simulink model "gm_ZynqBF_2tx_fpga"  (R2018b)
settings: Solver=FixedStepDiscrete  StartTime=0.0  StopTime=10.0  FixedStep=(1/420e3)/128  RelTol=1e-3
undefined symbols (not defined in the file or in its folder): a, b, c
libraries: hdlsllib x873, simulink x349
(part 7 of 40)

== system gm_ZynqBF_2tx_fpga/channel_estimator/peakdetect_ch2/peak_fsm ==
  t_cross : Inport  OutDataTypeStr=boolean  PortDimensions=1  SampleTime=1.86011904761905e-08
  cnt_end : Inport  Port=2  OutDataTypeStr=boolean  PortDimensions=1  SampleTime=1.86011904761905e-08
  Compare To Constant : simulink/Logic and Bit Operations/Compare To Constant  relop===  const=fi(0,0,8,0,'hex','01')  OutDataTypeStr=boolean
  Compare To Constant1 : simulink/Logic and Bit Operations/Compare To Constant  relop===  const=fi(0,0,8,0,'hex','00')  OutDataTypeStr=boolean
  Compare To Constant2 : simulink/Logic and Bit Operations/Compare To Constant  relop===  const=fi(0,0,8,0,'hex','02')  OutDataTypeStr=boolean
  HDL Counter : hdlsllib/Sources/HDL Counter  CountType=Count limited  CountInit=double(0)  CountStep=double(1)  CountMax=double(3)  CountFromType=Initial value  CountFrom=double(0)  CountResetPort=off  CountLoadPort=off  CountEnbPort=on  CountDirPort=off  CountDataType=Unsigned  CountWordLen=8  CountFracLen=0  CountSampTime=1.86011904761905e-08
      settings: SourceProductBaseCode=HD
  Logical Operator : Logic  AllPortsSameDT=off  OutDataTypeStr=boolean  SampleTime=1.86011904761905e-08
  Logical Operator1 : Logic  Operator=OR  Inputs=3  AllPortsSameDT=off  OutDataTypeStr=boolean  SampleTime=1.86011904761905e-08
  scan_peak : Outport
  peak_found : Outport  Port=2
  wires:
  t_cross/1 -> Logical Operator/1
  cnt_end/1 -> Logical Operator1/2
  Compare To Constant/1 -> scan_peak/1
  Compare To Constant1/1 -> Logical Operator/2
  Compare To Constant2/1 -> Logical Operator1/1, peak_found/1
  HDL Counter/1 -> Compare To Constant2/1, Compare To Constant1/1, Compare To Constant/1
  Logical Operator/1 -> Logical Operator1/3
  Logical Operator1/1 -> HDL Counter/1

== system gm_ZynqBF_2tx_fpga/channel_estimator/peakdetect_ch2/running_max ==
  din : Inport  OutDataTypeStr=fixdt(1, 32, 16)  PortDimensions=1  SampleTime=1.86011904761905e-08
  en : Inport  Port=2  OutDataTypeStr=boolean  PortDimensions=1  SampleTime=1.86011904761905e-08
  rst : Inport  Port=3  OutDataTypeStr=boolean  PortDimensions=1  SampleTime=1.86011904761905e-08
  Constant : Constant  Value=0  OutDataTypeStr=fixdt(1, 32, 16)  SampleTime=-1
  Delay4 : Delay  DelayLength=double(1)  InitialCondition=0  InputProcessing=Inherited  SampleTime=1.86011904761905e-08
  Relational Operator : RelationalOperator  Operator=>  OutDataTypeStr=boolean  SampleTime=1.86011904761905e-08  RndMeth=Nearest
  reset_max : Switch  Criteria=u2 ~= 0  Threshold=double(0)  OutDataTypeStr=fixdt(1, 32, 16)  SampleTime=1.86011904761905e-08
  store_max : Switch  Criteria=u2 ~= 0  Threshold=double(0)  OutDataTypeStr=fixdt(1, 32, 16)  SampleTime=1.86011904761905e-08
  update_max : Logic  AllPortsSameDT=off  OutDataTypeStr=boolean  SampleTime=1.86011904761905e-08
  new_max : Outport
  max_val : Outport  Port=2
  wires:
  din/1 -> store_max/1, Relational Operator/1
  en/1 -> update_max/1
  rst/1 -> reset_max/2
  Constant/1 -> reset_max/1
  Delay4/1 -> store_max/3, Relational Operator/2, max_val/1
  Relational Operator/1 -> update_max/2
  reset_max/1 -> Delay4/1
  store_max/1 -> reset_max/3
  update_max/1 -> store_max/2, new_max/1

== system gm_ZynqBF_2tx_fpga/channel_estimator/peakdetect_ch2/store_index ==
  din : Inport  OutDataTypeStr=int16  PortDimensions=1  SampleTime=1.86011904761905e-08
  update : Inport  Port=2  OutDataTypeStr=boolean  PortDimensions=1  SampleTime=1.86011904761905e-08
  Delay{1..2,4..5} (4 alike) : Delay  DelayLength=double(1)  InitialCondition=0  InputProcessing=Inherited  SampleTime=1.86011904761905e-08
  Switch : Switch  Criteria=u2 ~= 0  Threshold=double(0)  OutDataTypeStr=int16  SampleTime=1.86011904761905e-08
  dout : Outport
  wires:
  din/1 -> Delay2/1
  update/1 -> Delay1/1
  Delay1/1 -> Switch/2
  Delay2/1 -> Switch/1
  Delay4/1 -> dout/1
  Delay5/1 -> Switch/3
  Switch/1 -> Delay5/1, Delay4/1

== system gm_ZynqBF_2tx_fpga/channel_estimator/ram_rd_counter/select_inputs ==
  en1 : Inport  OutDataTypeStr=boolean  PortDimensions=1  SampleTime=1.86011904761905e-08
  en2 : Inport  Port=2  OutDataTypeStr=boolean  PortDimensions=1  SampleTime=1.86011904761905e-08
  in1 : Inport  Port=3  OutDataTypeStr=fixdt(0, 15, 0)  PortDimensions=1  SampleTime=1.86011904761905e-08
  in2 : Inport  Port=4  OutDataTypeStr=fixdt(0, 15, 0)  PortDimensions=1  SampleTime=1.86011904761905e-08
  select_inputs : MATLAB Function  TreatAsAtomicUnit=on
  y : Outport
  wires:
  en1/1 -> select_inputs/1(en1)
  en2/1 -> select_inputs/2(en2)
  in1/1 -> select_inputs/3(in1)
  in2/1 -> select_inputs/4(in2)
  select_inputs/1(y) -> y/1

== system gm_ZynqBF_2tx_fpga/channel_estimator/ch_est/calc_inverse/HDL Reciprocal ==
  In1 : Inport
  Delay1 : Delay  DelayLength=1  InputProcessing=Inherited
  Delay2 : Delay  DelayLength=10  InputProcessing=Inherited
  HDL Reciprocal : Reciprocal  NumberOfIterations=5  SampleTime=1.86011904761905e-08
  Out1 : Outport
  wires:
  In1/1 -> Delay1/1
  Delay1/1 -> HDL Reciprocal/1
  HDL Reciprocal/1 -> Delay2/1
  Delay2/1 -> Out1/1

== system gm_ZynqBF_2tx_fpga/channel_estimator/peakdetect_ch1/correlator1/all_u ==
  u : Inport  OutDataTypeStr=boolean  PortDimensions=[8]  SampleTime=1.86011904761905e-08
  all_u : MATLAB Function  TreatAsAtomicUnit=on
  y : Outport
  wires:
  u/1 -> all_u/1(u)
  all_u/1(y) -> y/1

== system gm_ZynqBF_2tx_fpga/channel_estimator/peakdetect_ch1/correlator1/all_u1 ==
  u : Inport  OutDataTypeStr=boolean  PortDimensions=[8]  SampleTime=1.86011904761905e-08
  all_u : MATLAB Function  TreatAsAtomicUnit=on
  y : Outport
  wires:
  all_u/1(y) -> y/1
  u/1 -> all_u/1(u)

== system gm_ZynqBF_2tx_fpga/channel_estimator/peakdetect_ch1/correlator1/correlation_config ==
  rst : Inport  OutDataTypeStr=boolean  PortDimensions=1  SampleTime=1.86011904761905e-08
  vin : Inport  Port=2  OutDataTypeStr=boolean  PortDimensions=1  SampleTime=1.86011904761905e-08
  Bit Slice : hdlsllib/Logic and Bit Operations/Bit Slice  lidx=double(14)  ridx=double(6)
  Delay{1..2,4..5} (4 alike) : Delay  DelayLength=double(1)  InitialCondition=0  InputProcessing=Inherited  SampleTime=1.86011904761905e-08
  Delay6 : Delay  DelayLength=double(3)  InitialCondition=0  InputProcessing=Inherited  SampleTime=1.86011904761905e-08
  correlation_count : hdlsllib/Sources/HDL Counter  CountType=Free running  CountInit=double(32767)  CountStep=double(1)  CountMax=25  CountFromType=Initial value  CountFrom=double(32767)  CountResetPort=on  CountLoadPort=off  CountEnbPort=on  CountDirPort=off  CountDataType=Unsigned  CountWordLen=15  CountFracLen=0  CountSampTime=1.86011904761905e-08
      settings: SourceProductBaseCode=HD
  shift_count : hdlsllib/Sources/HDL Counter  CountType=Free running  CountInit=double(63)  CountStep=double(1)  CountMax=25  CountFromType=Initial value  CountFrom=double(63)  CountResetPort=on  CountLoadPort=off  CountEnbPort=on  CountDirPort=off  CountDataType=Unsigned  CountWordLen=6  CountFracLen=0  CountSampTime=1.86011904761905e-08
      settings: SourceProductBaseCode=HD
  addr : Outport
  shift : Outport  Port=2
  vout : Outport  Port=3
  wires:
  rst/1 -> Delay4/1
  vin/1 -> Delay1/1
  Bit Slice/1 -> Delay2/1
  Delay1/1 -> shift_count/2, correlation_count/2, Delay6/1
  Delay2/1 -> addr/1
  Delay4/1 -> shift_count/1, correlation_count/1
  Delay5/1 -> shift/1
  Delay6/1 -> vout/1
  correlation_count/1 -> Bit Slice/1
  shift_count/1 -> Delay5/1

== system gm_ZynqBF_2tx_fpga/channel_estimator/peakdetect_ch1/correlator1/correlator_en ==
  valid : Inport  OutDataTypeStr=boolean  PortDimensions=1  SampleTime=1.86011904761905e-08
  done : Inport  Port=2  OutDataTypeStr=boolean  PortDimensions=1  SampleTime=1.86011904761905e-08
  addri : Inport  Port=3  OutDataTypeStr=fixdt(0, 9, 0)  PortDimensions=1  SampleTime=1.86011904761905e-08
  Compare To Constant : simulink/Logic and Bit Operations/Compare To Constant  relop===  const=fi(0,0,6,0,'hex','01')  OutDataTypeStr=boolean
  Delay1 : Delay  DelayLength=double(1)  InitialCondition=0  InputProcessing=Inherited  SampleTime=1.86011904761905e-08
  Delay2 : Delay  DelayLength=double(1)  InitialCondition=0  InputProcessing=Inherited  SampleTime=1.86011904761905e-08
  Delay3 : Delay  DelayLength=double(1)  InitialCondition=0  InputProcessing=Inherited  SampleTime=1.86011904761905e-08
  Sum : Sum  AccumDataTypeStr=fixdt(0, 10, 0)  OutDataTypeStr=fixdt(0, 10, 0)  SampleTime=1.86011904761905e-08
  corr_addr : hdlsllib/Sources/HDL Counter  CountType=Count limited  CountInit=double(0)  CountStep=double(1)  CountMax=double(63)  CountFromType=Initial value  CountFrom=double(0)  CountResetPort=on  CountLoadPort=off  CountEnbPort=on  CountDirPort=off  CountDataType=Unsigned  CountWordLen=6  CountFracLen=0  CountSampTime=1.86011904761905e-08
      settings: SourceProductBaseCode=HD
  corr_state : hdlsllib/Sources/HDL Counter  CountType=Count limited  CountInit=double(0)  CountStep=double(1)  CountMax=double(1)  CountFromType=Initial value  CountFrom=double(0)  CountResetPort=on  CountLoadPort=off  CountEnbPort=on  CountDirPort=off  CountDataType=Unsigned  CountWordLen=6  CountFracLen=0  CountSampTime=1.86011904761905e-08
      settings: SourceProductBaseCode=HD
  start : Outport
  en : Outport  Port=2
  gs_addr : Outport  Port=3
  rx_addr : Outport  Port=4
  wires:
  valid/1 -> corr_addr/1, Delay1/1
  done/1 -> corr_state/1
  addri/1 -> Sum/2
  Compare To Constant/1 -> Delay2/1
  Delay1/1 -> corr_state/2, Delay3/1
  Delay2/1 -> corr_addr/2, en/1
  Delay3/1 -> start/1
  Sum/1 -> rx_addr/1
  corr_addr/1 -> Sum/1, gs_addr/1
  corr_state/1 -> Compare To Constant/1

== system gm_ZynqBF_2tx_fpga/channel_estimator/peakdetect_ch1/correlator1/correlator_i_instance1 ==
  rx : Inport  OutDataTypeStr=fixdt(1, 16, 15)  PortDimensions=1  SampleTime=1.86011904761905e-08
  gs : Inport  Port=2  OutDataTypeStr=fixdt(1, 16, 15)  PortDimensions=1  SampleTime=1.86011904761905e-08
  start : Inport  Port=3  OutDataTypeStr=boolean  PortDimensions=1  SampleTime=1.86011904761905e-08
  vin : Inport  Port=4  OutDataTypeStr=boolean  PortDimensions=1  SampleTime=1.86011904761905e-08
  Compare To Constant1 : simulink/Logic and Bit Operations/Compare To Constant  relop===  const=fi(0,0,7,0,'hex','3f')  OutDataTypeStr=boolean
  Constant : Constant  Value=0  OutDataTypeStr=fixdt(1, 32, 16)  SampleTime=-1
  Constant1 : Constant  Value=0  OutDataTypeStr=fixdt(1, 16, 15)  SampleTime=-1
  Delay1 : Delay  DelayLength=double(1)  InitialCondition=0  InputProcessing=Inherited  SampleTime=1.86011904761905e-08
  HDL Counter : hdlsllib/Sources/HDL Counter  CountType=Free running  CountInit=double(0)  CountStep=double(1)  CountMax=25  CountFromType=Initial value  CountFrom=double(0)  CountResetPort=on  CountLoadPort=off  CountEnbPort=on  CountDirPort=off  CountDataType=Unsigned  CountWordLen=7  CountFracLen=0  CountSampTime=1.86011904761905e-08
      settings: SourceProductBaseCode=HD
  Multiply-Add : hdlsllib/HDL Operations/Multiply-Add  Function=c+(a.*b)  datatype=fixdt(1, 32, 16)  DoSatur=off  FMA=off
      settings: SourceProductName=HDL Coder  SourceProductBaseCode=HD
  Switch : Switch  Criteria=u2 ~= 0  Threshold=double(0)  OutDataTypeStr=fixdt(1, 32, 16)  SampleTime=1.86011904761905e-08
  Switch1 : Switch  Criteria=u2 ~= 0  Threshold=double(0)  OutDataTypeStr=fixdt(1, 16, 15)  SampleTime=1.86011904761905e-08
  Switch2 : Switch  Criteria=u2 ~= 0  Threshold=double(0)  OutDataTypeStr=fixdt(1, 16, 15)  SampleTime=1.86011904761905e-08
  dout : Outport
  vout : Outport  Port=2
  wires:
  Switch2/1 -> Multiply-Add/2
  Switch1/1 -> Multiply-Add/1
  Multiply-Add/1 -> dout/1, Delay1/1
  HDL Counter/1 -> Compare To Constant1/1
  Constant1/1 -> Switch1/3, Switch2/3
  Constant/1 -> Switch/1
  Compare To Constant1/1 -> vout/1
  rx/1 -> Switch1/1
  gs/1 -> Switch2/1
  start/1 -> HDL Counter/1, Switch/2
  vin/1 -> Switch1/2, Switch2/2, HDL Counter/2
  Delay1/1 -> Switch/3
  Switch/1 -> Multiply-Add/3

== system gm_ZynqBF_2tx_fpga/channel_estimator/peakdetect_ch1/correlator1/correlator_i_instance10 ==
  rx : Inport  OutDataTypeStr=fixdt(1, 16, 15)  PortDimensions=1  SampleTime=1.86011904761905e-08
  gs : Inport  Port=2  OutDataTypeStr=fixdt(1, 16, 15)  PortDimensions=1  SampleTime=1.86011904761905e-08
  start : Inport  Port=3  OutDataTypeStr=boolean  PortDimensions=1  SampleTime=1.86011904761905e-08
  vin : Inport  Port=4  OutDataTypeStr=boolean  PortDimensions=1  SampleTime=1.86011904761905e-08
  Compare To Constant1 : simulink/Logic and Bit Operations/Compare To Constant  relop===  const=fi(0,0,7,0,'hex','3f')  OutDataTypeStr=boolean
  Constant : Constant  Value=0  OutDataTypeStr=fixdt(1, 32, 16)  SampleTime=-1
  Constant1 : Constant  Value=0  OutDataTypeStr=fixdt(1, 16, 15)  SampleTime=-1
  Delay1 : Delay  DelayLength=double(1)  InitialCondition=0  InputProcessing=Inherited  SampleTime=1.86011904761905e-08
  HDL Counter : hdlsllib/Sources/HDL Counter  CountType=Free running  CountInit=double(0)  CountStep=double(1)  CountMax=25  CountFromType=Initial value  CountFrom=double(0)  CountResetPort=on  CountLoadPort=off  CountEnbPort=on  CountDirPort=off  CountDataType=Unsigned  CountWordLen=7  CountFracLen=0  CountSampTime=1.86011904761905e-08
      settings: SourceProductBaseCode=HD
  Multiply-Add : hdlsllib/HDL Operations/Multiply-Add  Function=c+(a.*b)  datatype=fixdt(1, 32, 16)  DoSatur=off  FMA=off
      settings: SourceProductName=HDL Coder  SourceProductBaseCode=HD
  Switch : Switch  Criteria=u2 ~= 0  Threshold=double(0)  OutDataTypeStr=fixdt(1, 32, 16)  SampleTime=1.86011904761905e-08
  Switch1 : Switch  Criteria=u2 ~= 0  Threshold=double(0)  OutDataTypeStr=fixdt(1, 16, 15)  SampleTime=1.86011904761905e-08
  Switch2 : Switch  Criteria=u2 ~= 0  Threshold=double(0)  OutDataTypeStr=fixdt(1, 16, 15)  SampleTime=1.86011904761905e-08
  dout : Outport
  vout : Outport  Port=2
  wires:
  Switch/1 -> Multiply-Add/3
  Delay1/1 -> Switch/3
  vin/1 -> HDL Counter/2, Switch2/2, Switch1/2
  start/1 -> Switch/2, HDL Counter/1
  gs/1 -> Switch2/1
  rx/1 -> Switch1/1
  Compare To Constant1/1 -> vout/1
  Constant/1 -> Switch/1
  Constant1/1 -> Switch2/3, Switch1/3
  HDL Counter/1 -> Compare To Constant1/1
  Multiply-Add/1 -> Delay1/1, dout/1
  Switch1/1 -> Multiply-Add/1
  Switch2/1 -> Multiply-Add/2

== system gm_ZynqBF_2tx_fpga/channel_estimator/peakdetect_ch1/correlator1/correlator_i_instance11 ==
  rx : Inport  OutDataTypeStr=fixdt(1, 16, 15)  PortDimensions=1  SampleTime=1.86011904761905e-08
  gs : Inport  Port=2  OutDataTypeStr=fixdt(1, 16, 15)  PortDimensions=1  SampleTime=1.86011904761905e-08
  start : Inport  Port=3  OutDataTypeStr=boolean  PortDimensions=1  SampleTime=1.86011904761905e-08
  vin : Inport  Port=4  OutDataTypeStr=boolean  PortDimensions=1  SampleTime=1.86011904761905e-08
  Compare To Constant1 : simulink/Logic and Bit Operations/Compare To Constant  relop===  const=fi(0,0,7,0,'hex','3f')  OutDataTypeStr=boolean
  Constant : Constant  Value=0  OutDataTypeStr=fixdt(1, 32, 16)  SampleTime=-1
  Constant1 : Constant  Value=0  OutDataTypeStr=fixdt(1, 16, 15)  SampleTime=-1
  Delay1 : Delay  DelayLength=double(1)  InitialCondition=0  InputProcessing=Inherited  SampleTime=1.86011904761905e-08
  HDL Counter : hdlsllib/Sources/HDL Counter  CountType=Free running  CountInit=double(0)  CountStep=double(1)  CountMax=25  CountFromType=Initial value  CountFrom=double(0)  CountResetPort=on  CountLoadPort=off  CountEnbPort=on  CountDirPort=off  CountDataType=Unsigned  CountWordLen=7  CountFracLen=0  CountSampTime=1.86011904761905e-08
      settings: SourceProductBaseCode=HD
  Multiply-Add : hdlsllib/HDL Operations/Multiply-Add  Function=c+(a.*b)  datatype=fixdt(1, 32, 16)  DoSatur=off  FMA=off
      settings: SourceProductName=HDL Coder  SourceProductBaseCode=HD
  Switch : Switch  Criteria=u2 ~= 0  Threshold=double(0)  OutDataTypeStr=fixdt(1, 32, 16)  SampleTime=1.86011904761905e-08
  Switch1 : Switch  Criteria=u2 ~= 0  Threshold=double(0)  OutDataTypeStr=fixdt(1, 16, 15)  SampleTime=1.86011904761905e-08
  Switch2 : Switch  Criteria=u2 ~= 0  Threshold=double(0)  OutDataTypeStr=fixdt(1, 16, 15)  SampleTime=1.86011904761905e-08
  dout : Outport
  vout : Outport  Port=2
  wires:
  Switch/1 -> Multiply-Add/3
  Delay1/1 -> Switch/3
  vin/1 -> HDL Counter/2, Switch2/2, Switch1/2
  start/1 -> Switch/2, HDL Counter/1
  gs/1 -> Switch2/1
  rx/1 -> Switch1/1
  Compare To Constant1/1 -> vout/1
  Constant/1 -> Switch/1
  Constant1/1 -> Switch2/3, Switch1/3
  HDL Counter/1 -> Compare To Constant1/1
  Multiply-Add/1 -> Delay1/1, dout/1
  Switch1/1 -> Multiply-Add/1
  Switch2/1 -> Multiply-Add/2

== system gm_ZynqBF_2tx_fpga/channel_estimator/peakdetect_ch1/correlator1/correlator_i_instance12 ==
  rx : Inport  OutDataTypeStr=fixdt(1, 16, 15)  PortDimensions=1  SampleTime=1.86011904761905e-08
  gs : Inport  Port=2  OutDataTypeStr=fixdt(1, 16, 15)  PortDimensions=1  SampleTime=1.86011904761905e-08
  start : Inport  Port=3  OutDataTypeStr=boolean  PortDimensions=1  SampleTime=1.86011904761905e-08
  vin : Inport  Port=4  OutDataTypeStr=boolean  PortDimensions=1  SampleTime=1.86011904761905e-08
  Compare To Constant1 : simulink/Logic and Bit Operations/Compare To Constant  relop===  const=fi(0,0,7,0,'hex','3f')  OutDataTypeStr=boolean
  Constant : Constant  Value=0  OutDataTypeStr=fixdt(1, 32, 16)  SampleTime=-1
  Constant1 : Constant  Value=0  OutDataTypeStr=fixdt(1, 16, 15)  SampleTime=-1
  Delay1 : Delay  DelayLength=double(1)  InitialCondition=0  InputProcessing=Inherited  SampleTime=1.86011904761905e-08
  HDL Counter : hdlsllib/Sources/HDL Counter  CountType=Free running  CountInit=double(0)  CountStep=double(1)  CountMax=25  CountFromType=Initial value  CountFrom=double(0)  CountResetPort=on  CountLoadPort=off  CountEnbPort=on  CountDirPort=off  CountDataType=Unsigned  CountWordLen=7  CountFracLen=0  CountSampTime=1.86011904761905e-08
      settings: SourceProductBaseCode=HD
  Multiply-Add : hdlsllib/HDL Operations/Multiply-Add  Function=c+(a.*b)  datatype=fixdt(1, 32, 16)  DoSatur=off  FMA=off
      settings: SourceProductName=HDL Coder  SourceProductBaseCode=HD
  Switch : Switch  Criteria=u2 ~= 0  Threshold=double(0)  OutDataTypeStr=fixdt(1, 32, 16)  SampleTime=1.86011904761905e-08
  Switch1 : Switch  Criteria=u2 ~= 0  Threshold=double(0)  OutDataTypeStr=fixdt(1, 16, 15)  SampleTime=1.86011904761905e-08
  Switch2 : Switch  Criteria=u2 ~= 0  Threshold=double(0)  OutDataTypeStr=fixdt(1, 16, 15)  SampleTime=1.86011904761905e-08
  dout : Outport
  vout : Outport  Port=2
  wires:
  Switch/1 -> Multiply-Add/3
  Delay1/1 -> Switch/3
  vin/1 -> HDL Counter/2, Switch2/2, Switch1/2
  start/1 -> Switch/2, HDL Counter/1
  gs/1 -> Switch2/1
  rx/1 -> Switch1/1
  Compare To Constant1/1 -> vout/1
  Constant/1 -> Switch/1
  Constant1/1 -> Switch2/3, Switch1/3
  HDL Counter/1 -> Compare To Constant1/1
  Multiply-Add/1 -> Delay1/1, dout/1
  Switch1/1 -> Multiply-Add/1
  Switch2/1 -> Multiply-Add/2

== system gm_ZynqBF_2tx_fpga/channel_estimator/peakdetect_ch1/correlator1/correlator_i_instance13 ==
  rx : Inport  OutDataTypeStr=fixdt(1, 16, 15)  PortDimensions=1  SampleTime=1.86011904761905e-08
  gs : Inport  Port=2  OutDataTypeStr=fixdt(1, 16, 15)  PortDimensions=1  SampleTime=1.86011904761905e-08
  start : Inport  Port=3  OutDataTypeStr=boolean  PortDimensions=1  SampleTime=1.86011904761905e-08
  vin : Inport  Port=4  OutDataTypeStr=boolean  PortDimensions=1  SampleTime=1.86011904761905e-08
  Compare To Constant1 : simulink/Logic and Bit Operations/Compare To Constant  relop===  const=fi(0,0,7,0,'hex','3f')  OutDataTypeStr=boolean
  Constant : Constant  Value=0  OutDataTypeStr=fixdt(1, 32, 16)  SampleTime=-1
  Constant1 : Constant  Value=0  OutDataTypeStr=fixdt(1, 16, 15)  SampleTime=-1
  Delay1 : Delay  DelayLength=double(1)  InitialCondition=0  InputProcessing=Inherited  SampleTime=1.86011904761905e-08
  HDL Counter : hdlsllib/Sources/HDL Counter  CountType=Free running  CountInit=double(0)  CountStep=double(1)  CountMax=25  CountFromType=Initial value  CountFrom=double(0)  CountResetPort=on  CountLoadPort=off  CountEnbPort=on  CountDirPort=off  CountDataType=Unsigned  CountWordLen=7  CountFracLen=0  CountSampTime=1.86011904761905e-08
      settings: SourceProductBaseCode=HD
  Multiply-Add : hdlsllib/HDL Operations/Multiply-Add  Function=c+(a.*b)  datatype=fixdt(1, 32, 16)  DoSatur=off  FMA=off
      settings: SourceProductName=HDL Coder  SourceProductBaseCode=HD
  Switch : Switch  Criteria=u2 ~= 0  Threshold=double(0)  OutDataTypeStr=fixdt(1, 32, 16)  SampleTime=1.86011904761905e-08
  Switch1 : Switch  Criteria=u2 ~= 0  Threshold=double(0)  OutDataTypeStr=fixdt(1, 16, 15)  SampleTime=1.86011904761905e-08
  Switch2 : Switch  Criteria=u2 ~= 0  Threshold=double(0)  OutDataTypeStr=fixdt(1, 16, 15)  SampleTime=1.86011904761905e-08
  dout : Outport
  vout : Outport  Port=2
  wires:
  Switch/1 -> Multiply-Add/3
  Delay1/1 -> Switch/3
  vin/1 -> HDL Counter/2, Switch2/2, Switch1/2
  start/1 -> Switch/2, HDL Counter/1
  gs/1 -> Switch2/1
  rx/1 -> Switch1/1
  Compare To Constant1/1 -> vout/1
  Constant/1 -> Switch/1
  Constant1/1 -> Switch2/3, Switch1/3
  HDL Counter/1 -> Compare To Constant1/1
  Multiply-Add/1 -> Delay1/1, dout/1
  Switch1/1 -> Multiply-Add/1
  Switch2/1 -> Multiply-Add/2

== system gm_ZynqBF_2tx_fpga/channel_estimator/peakdetect_ch1/correlator1/correlator_i_instance14 ==
  rx : Inport  OutDataTypeStr=fixdt(1, 16, 15)  PortDimensions=1  SampleTime=1.86011904761905e-08
  gs : Inport  Port=2  OutDataTypeStr=fixdt(1, 16, 15)  PortDimensions=1  SampleTime=1.86011904761905e-08
  start : Inport  Port=3  OutDataTypeStr=boolean  PortDimensions=1  SampleTime=1.86011904761905e-08
  vin : Inport  Port=4  OutDataTypeStr=boolean  PortDimensions=1  SampleTime=1.86011904761905e-08
  Compare To Constant1 : simulink/Logic and Bit Operations/Compare To Constant  relop===  const=fi(0,0,7,0,'hex','3f')  OutDataTypeStr=boolean
  Constant : Constant  Value=0  OutDataTypeStr=fixdt(1, 32, 16)  SampleTime=-1
  Constant1 : Constant  Value=0  OutDataTypeStr=fixdt(1, 16, 15)  SampleTime=-1
  Delay1 : Delay  DelayLength=double(1)  InitialCondition=0  InputProcessing=Inherited  SampleTime=1.86011904761905e-08
  HDL Counter : hdlsllib/Sources/HDL Counter  CountType=Free running  CountInit=double(0)  CountStep=double(1)  CountMax=25  CountFromType=Initial value  CountFrom=double(0)  CountResetPort=on  CountLoadPort=off  CountEnbPort=on  CountDirPort=off  CountDataType=Unsigned  CountWordLen=7  CountFracLen=0  CountSampTime=1.86011904761905e-08
      settings: SourceProductBaseCode=HD
  Multiply-Add : hdlsllib/HDL Operations/Multiply-Add  Function=c+(a.*b)  datatype=fixdt(1, 32, 16)  DoSatur=off  FMA=off
      settings: SourceProductName=HDL Coder  SourceProductBaseCode=HD
  Switch : Switch  Criteria=u2 ~= 0  Threshold=double(0)  OutDataTypeStr=fixdt(1, 32, 16)  SampleTime=1.86011904761905e-08
  Switch1 : Switch  Criteria=u2 ~= 0  Threshold=double(0)  OutDataTypeStr=fixdt(1, 16, 15)  SampleTime=1.86011904761905e-08
  Switch2 : Switch  Criteria=u2 ~= 0  Threshold=double(0)  OutDataTypeStr=fixdt(1, 16, 15)  SampleTime=1.86011904761905e-08
  dout : Outport
  vout : Outport  Port=2
  wires:
  Switch/1 -> Multiply-Add/3
  Delay1/1 -> Switch/3
  vin/1 -> HDL Counter/2, Switch2/2, Switch1/2
  start/1 -> Switch/2, HDL Counter/1
  gs/1 -> Switch2/1
  rx/1 -> Switch1/1
  Compare To Constant1/1 -> vout/1
  Constant/1 -> Switch/1
  Constant1/1 -> Switch2/3, Switch1/3
  HDL Counter/1 -> Compare To Constant1/1
  Multiply-Add/1 -> Delay1/1, dout/1
  Switch1/1 -> Multiply-Add/1
  Switch2/1 -> Multiply-Add/2

== system gm_ZynqBF_2tx_fpga/channel_estimator/peakdetect_ch1/correlator1/correlator_i_instance15 ==
  rx : Inport  OutDataTypeStr=fixdt(1, 16, 15)  PortDimensions=1  SampleTime=1.86011904761905e-08
  gs : Inport  Port=2  OutDataTypeStr=fixdt(1, 16, 15)  PortDimensions=1  SampleTime=1.86011904761905e-08
  start : Inport  Port=3  OutDataTypeStr=boolean  PortDimensions=1  SampleTime=1.86011904761905e-08
  vin : Inport  Port=4  OutDataTypeStr=boolean  PortDimensions=1  SampleTime=1.86011904761905e-08
  Compare To Constant1 : simulink/Logic and Bit Operations/Compare To Constant  relop===  const=fi(0,0,7,0,'hex','3f')  OutDataTypeStr=boolean
  Constant : Constant  Value=0  OutDataTypeStr=fixdt(1, 32, 16)  SampleTime=-1
  Constant1 : Constant  Value=0  OutDataTypeStr=fixdt(1, 16, 15)  SampleTime=-1
  Delay1 : Delay  DelayLength=double(1)  InitialCondition=0  InputProcessing=Inherited  SampleTime=1.86011904761905e-08
  HDL Counter : hdlsllib/Sources/HDL Counter  CountType=Free running  CountInit=double(0)  CountStep=double(1)  CountMax=25  CountFromType=Initial value  CountFrom=double(0)  CountResetPort=on  CountLoadPort=off  CountEnbPort=on  CountDirPort=off  CountDataType=Unsigned  CountWordLen=7  CountFracLen=0  CountSampTime=1.86011904761905e-08
      settings: SourceProductBaseCode=HD
  Multiply-Add : hdlsllib/HDL Operations/Multiply-Add  Function=c+(a.*b)  datatype=fixdt(1, 32, 16)  DoSatur=off  FMA=off
      settings: SourceProductName=HDL Coder  SourceProductBaseCode=HD
  Switch : Switch  Criteria=u2 ~= 0  Threshold=double(0)  OutDataTypeStr=fixdt(1, 32, 16)  SampleTime=1.86011904761905e-08
  Switch1 : Switch  Criteria=u2 ~= 0  Threshold=double(0)  OutDataTypeStr=fixdt(1, 16, 15)  SampleTime=1.86011904761905e-08
  Switch2 : Switch  Criteria=u2 ~= 0  Threshold=double(0)  OutDataTypeStr=fixdt(1, 16, 15)  SampleTime=1.86011904761905e-08
  dout : Outport
  vout : Outport  Port=2
  wires:
  Switch/1 -> Multiply-Add/3
  Delay1/1 -> Switch/3
  vin/1 -> HDL Counter/2, Switch2/2, Switch1/2
  start/1 -> Switch/2, HDL Counter/1
  gs/1 -> Switch2/1
  rx/1 -> Switch1/1
  Compare To Constant1/1 -> vout/1
  Constant/1 -> Switch/1
  Constant1/1 -> Switch2/3, Switch1/3
  HDL Counter/1 -> Compare To Constant1/1
  Multiply-Add/1 -> Delay1/1, dout/1
  Switch1/1 -> Multiply-Add/1
  Switch2/1 -> Multiply-Add/2

== system gm_ZynqBF_2tx_fpga/channel_estimator/peakdetect_ch1/correlator1/correlator_i_instance16 ==
  rx : Inport  OutDataTypeStr=fixdt(1, 16, 15)  PortDimensions=1  SampleTime=1.86011904761905e-08
  gs : Inport  Port=2  OutDataTypeStr=fixdt(1, 16, 15)  PortDimensions=1  SampleTime=1.86011904761905e-08
  start : Inport  Port=3  OutDataTypeStr=boolean  PortDimensions=1  SampleTime=1.86011904761905e-08
  vin : Inport  Port=4  OutDataTypeStr=boolean  PortDimensions=1  SampleTime=1.86011904761905e-08
  Compare To Constant1 : simulink/Logic and Bit Operations/Compare To Constant  relop===  const=fi(0,0,7,0,'hex','3f')  OutDataTypeStr=boolean
  Constant : Constant  Value=0  OutDataTypeStr=fixdt(1, 32, 16)  SampleTime=-1
  Constant1 : Constant  Value=0  OutDataTypeStr=fixdt(1, 16, 15)  SampleTime=-1
  Delay1 : Delay  DelayLength=double(1)  InitialCondition=0  InputProcessing=Inherited  SampleTime=1.86011904761905e-08
  HDL Counter : hdlsllib/Sources/HDL Counter  CountType=Free running  CountInit=double(0)  CountStep=double(1)  CountMax=25  CountFromType=Initial value  CountFrom=double(0)  CountResetPort=on  CountLoadPort=off  CountEnbPort=on  CountDirPort=off  CountDataType=Unsigned  CountWordLen=7  CountFracLen=0  CountSampTime=1.86011904761905e-08
      settings: SourceProductBaseCode=HD
  Multiply-Add : hdlsllib/HDL Operations/Multiply-Add  Function=c+(a.*b)  datatype=fixdt(1, 32, 16)  DoSatur=off  FMA=off
      settings: SourceProductName=HDL Coder  SourceProductBaseCode=HD
  Switch : Switch  Criteria=u2 ~= 0  Threshold=double(0)  OutDataTypeStr=fixdt(1, 32, 16)  SampleTime=1.86011904761905e-08
  Switch1 : Switch  Criteria=u2 ~= 0  Threshold=double(0)  OutDataTypeStr=fixdt(1, 16, 15)  SampleTime=1.86011904761905e-08
  Switch2 : Switch  Criteria=u2 ~= 0  Threshold=double(0)  OutDataTypeStr=fixdt(1, 16, 15)  SampleTime=1.86011904761905e-08
  dout : Outport
  vout : Outport  Port=2
  wires:
  Switch/1 -> Multiply-Add/3
  Delay1/1 -> Switch/3
  vin/1 -> HDL Counter/2, Switch2/2, Switch1/2
  start/1 -> Switch/2, HDL Counter/1
  gs/1 -> Switch2/1
  rx/1 -> Switch1/1
  Compare To Constant1/1 -> vout/1
  Constant/1 -> Switch/1
  Constant1/1 -> Switch2/3, Switch1/3
  HDL Counter/1 -> Compare To Constant1/1
  Multiply-Add/1 -> Delay1/1, dout/1
  Switch1/1 -> Multiply-Add/1
  Switch2/1 -> Multiply-Add/2

== system gm_ZynqBF_2tx_fpga/channel_estimator/peakdetect_ch1/correlator1/correlator_i_instance17 ==
  rx : Inport  OutDataTypeStr=fixdt(1, 16, 15)  PortDimensions=1  SampleTime=1.86011904761905e-08
  gs : Inport  Port=2  OutDataTypeStr=fixdt(1, 16, 15)  PortDimensions=1  SampleTime=1.86011904761905e-08
  start : Inport  Port=3  OutDataTypeStr=boolean  PortDimensions=1  SampleTime=1.86011904761905e-08
  vin : Inport  Port=4  OutDataTypeStr=boolean  PortDimensions=1  SampleTime=1.86011904761905e-08
  Compare To Constant1 : simulink/Logic and Bit Operations/Compare To Constant  relop===  const=fi(0,0,7,0,'hex','3f')  OutDataTypeStr=boolean
  Constant : Constant  Value=0  OutDataTypeStr=fixdt(1, 32, 16)  SampleTime=-1
  Constant1 : Constant  Value=0  OutDataTypeStr=fixdt(1, 16, 15)  SampleTime=-1
  Delay1 : Delay  DelayLength=double(1)  InitialCondition=0  InputProcessing=Inherited  SampleTime=1.86011904761905e-08
  HDL Counter : hdlsllib/Sources/HDL Counter  CountType=Free running  CountInit=double(0)  CountStep=double(1)  CountMax=25  CountFromType=Initial value  CountFrom=double(0)  CountResetPort=on  CountLoadPort=off  CountEnbPort=on  CountDirPort=off  CountDataType=Unsigned  CountWordLen=7  CountFracLen=0  CountSampTime=1.86011904761905e-08
      settings: SourceProductBaseCode=HD
  Multiply-Add : hdlsllib/HDL Operations/Multiply-Add  Function=c+(a.*b)  datatype=fixdt(1, 32, 16)  DoSatur=off  FMA=off
      settings: SourceProductName=HDL Coder  SourceProductBaseCode=HD
  Switch : Switch  Criteria=u2 ~= 0  Threshold=double(0)  OutDataTypeStr=fixdt(1, 32, 16)  SampleTime=1.86011904761905e-08
  Switch1 : Switch  Criteria=u2 ~= 0  Threshold=double(0)  OutDataTypeStr=fixdt(1, 16, 15)  SampleTime=1.86011904761905e-08
  Switch2 : Switch  Criteria=u2 ~= 0  Threshold=double(0)  OutDataTypeStr=fixdt(1, 16, 15)  SampleTime=1.86011904761905e-08
  dout : Outport
  vout : Outport  Port=2
  wires:
  Switch/1 -> Multiply-Add/3
  Delay1/1 -> Switch/3
  vin/1 -> HDL Counter/2, Switch2/2, Switch1/2
  start/1 -> Switch/2, HDL Counter/1
  gs/1 -> Switch2/1
  rx/1 -> Switch1/1
  Compare To Constant1/1 -> vout/1
  Constant/1 -> Switch/1
  Constant1/1 -> Switch2/3, Switch1/3
  HDL Counter/1 -> Compare To Constant1/1
  Multiply-Add/1 -> Delay1/1, dout/1
  Switch1/1 -> Multiply-Add/1
  Switch2/1 -> Multiply-Add/2

== system gm_ZynqBF_2tx_fpga/channel_estimator/peakdetect_ch1/correlator1/correlator_i_instance18 ==
  rx : Inport  OutDataTypeStr=fixdt(1, 16, 15)  PortDimensions=1  SampleTime=1.86011904761905e-08
  gs : Inport  Port=2  OutDataTypeStr=fixdt(1, 16, 15)  PortDimensions=1  SampleTime=1.86011904761905e-08
  start : Inport  Port=3  OutDataTypeStr=boolean  PortDimensions=1  SampleTime=1.86011904761905e-08
  vin : Inport  Port=4  OutDataTypeStr=boolean  PortDimensions=1  SampleTime=1.86011904761905e-08
  Compare To Constant1 : simulink/Logic and Bit Operations/Compare To Constant  relop===  const=fi(0,0,7,0,'hex','3f')  OutDataTypeStr=boolean
  Constant : Constant  Value=0  OutDataTypeStr=fixdt(1, 32, 16)  SampleTime=-1
  Constant1 : Constant  Value=0  OutDataTypeStr=fixdt(1, 16, 15)  SampleTime=-1
  Delay1 : Delay  DelayLength=double(1)  InitialCondition=0  InputProcessing=Inherited  SampleTime=1.86011904761905e-08
  HDL Counter : hdlsllib/Sources/HDL Counter  CountType=Free running  CountInit=double(0)  CountStep=double(1)  CountMax=25  CountFromType=Initial value  CountFrom=double(0)  CountResetPort=on  CountLoadPort=off  CountEnbPort=on  CountDirPort=off  CountDataType=Unsigned  CountWordLen=7  CountFracLen=0  CountSampTime=1.86011904761905e-08
      settings: SourceProductBaseCode=HD
  Multiply-Add : hdlsllib/HDL Operations/Multiply-Add  Function=c+(a.*b)  datatype=fixdt(1, 32, 16)  DoSatur=off  FMA=off
      settings: SourceProductName=HDL Coder  SourceProductBaseCode=HD
  Switch : Switch  Criteria=u2 ~= 0  Threshold=double(0)  OutDataTypeStr=fixdt(1, 32, 16)  SampleTime=1.86011904761905e-08
  Switch1 : Switch  Criteria=u2 ~= 0  Threshold=double(0)  OutDataTypeStr=fixdt(1, 16, 15)  SampleTime=1.86011904761905e-08
  Switch2 : Switch  Criteria=u2 ~= 0  Threshold=double(0)  OutDataTypeStr=fixdt(1, 16, 15)  SampleTime=1.86011904761905e-08
  dout : Outport
  vout : Outport  Port=2
  wires:
  Switch/1 -> Multiply-Add/3
  Delay1/1 -> Switch/3
  vin/1 -> HDL Counter/2, Switch2/2, Switch1/2
  start/1 -> Switch/2, HDL Counter/1
  gs/1 -> Switch2/1
  rx/1 -> Switch1/1
  Compare To Constant1/1 -> vout/1
  Constant/1 -> Switch/1
  Constant1/1 -> Switch2/3, Switch1/3
  HDL Counter/1 -> Compare To Constant1/1
  Multiply-Add/1 -> Delay1/1, dout/1
  Switch1/1 -> Multiply-Add/1
  Switch2/1 -> Multiply-Add/2

== system gm_ZynqBF_2tx_fpga/channel_estimator/peakdetect_ch1/correlator1/correlator_i_instance19 ==
  rx : Inport  OutDataTypeStr=fixdt(1, 16, 15)  PortDimensions=1  SampleTime=1.86011904761905e-08
  gs : Inport  Port=2  OutDataTypeStr=fixdt(1, 16, 15)  PortDimensions=1  SampleTime=1.86011904761905e-08
  start : Inport  Port=3  OutDataTypeStr=boolean  PortDimensions=1  SampleTime=1.86011904761905e-08
  vin : Inport  Port=4  OutDataTypeStr=boolean  PortDimensions=1  SampleTime=1.86011904761905e-08
  Compare To Constant1 : simulink/Logic and Bit Operations/Compare To Constant  relop===  const=fi(0,0,7,0,'hex','3f')  OutDataTypeStr=boolean
  Constant : Constant  Value=0  OutDataTypeStr=fixdt(1, 32, 16)  SampleTime=-1
  Constant1 : Constant  Value=0  OutDataTypeStr=fixdt(1, 16, 15)  SampleTime=-1
  Delay1 : Delay  DelayLength=double(1)  InitialCondition=0  InputProcessing=Inherited  SampleTime=1.86011904761905e-08
  HDL Counter : hdlsllib/Sources/HDL Counter  CountType=Free running  CountInit=double(0)  CountStep=double(1)  CountMax=25  CountFromType=Initial value  CountFrom=double(0)  CountResetPort=on  CountLoadPort=off  CountEnbPort=on  CountDirPort=off  CountDataType=Unsigned  CountWordLen=7  CountFracLen=0  CountSampTime=1.86011904761905e-08
      settings: SourceProductBaseCode=HD
  Multiply-Add : hdlsllib/HDL Operations/Multiply-Add  Function=c+(a.*b)  datatype=fixdt(1, 32, 16)  DoSatur=off  FMA=off
      settings: SourceProductName=HDL Coder  SourceProductBaseCode=HD
  Switch : Switch  Criteria=u2 ~= 0  Threshold=double(0)  OutDataTypeStr=fixdt(1, 32, 16)  SampleTime=1.86011904761905e-08
  Switch1 : Switch  Criteria=u2 ~= 0  Threshold=double(0)  OutDataTypeStr=fixdt(1, 16, 15)  SampleTime=1.86011904761905e-08
  Switch2 : Switch  Criteria=u2 ~= 0  Threshold=double(0)  OutDataTypeStr=fixdt(1, 16, 15)  SampleTime=1.86011904761905e-08
  dout : Outport
  vout : Outport  Port=2
  wires:
  Switch/1 -> Multiply-Add/3
  Delay1/1 -> Switch/3
  vin/1 -> HDL Counter/2, Switch2/2, Switch1/2
  start/1 -> Switch/2, HDL Counter/1
  gs/1 -> Switch2/1
  rx/1 -> Switch1/1
  Compare To Constant1/1 -> vout/1
  Constant/1 -> Switch/1
  Constant1/1 -> Switch2/3, Switch1/3
  HDL Counter/1 -> Compare To Constant1/1
  Multiply-Add/1 -> Delay1/1, dout/1
  Switch1/1 -> Multiply-Add/1
  Switch2/1 -> Multiply-Add/2

== system gm_ZynqBF_2tx_fpga/channel_estimator/peakdetect_ch1/correlator1/correlator_i_instance2 ==
  rx : Inport  OutDataTypeStr=fixdt(1, 16, 15)  PortDimensions=1  SampleTime=1.86011904761905e-08
  gs : Inport  Port=2  OutDataTypeStr=fixdt(1, 16, 15)  PortDimensions=1  SampleTime=1.86011904761905e-08
  start : Inport  Port=3  OutDataTypeStr=boolean  PortDimensions=1  SampleTime=1.86011904761905e-08
  vin : Inport  Port=4  OutDataTypeStr=boolean  PortDimensions=1  SampleTime=1.86011904761905e-08
  Compare To Constant1 : simulink/Logic and Bit Operations/Compare To Constant  relop===  const=fi(0,0,7,0,'hex','3f')  OutDataTypeStr=boolean
  Constant : Constant  Value=0  OutDataTypeStr=fixdt(1, 32, 16)  SampleTime=-1
  Constant1 : Constant  Value=0  OutDataTypeStr=fixdt(1, 16, 15)  SampleTime=-1
  Delay1 : Delay  DelayLength=double(1)  InitialCondition=0  InputProcessing=Inherited  SampleTime=1.86011904761905e-08
  HDL Counter : hdlsllib/Sources/HDL Counter  CountType=Free running  CountInit=double(0)  CountStep=double(1)  CountMax=25  CountFromType=Initial value  CountFrom=double(0)  CountResetPort=on  CountLoadPort=off  CountEnbPort=on  CountDirPort=off  CountDataType=Unsigned  CountWordLen=7  CountFracLen=0  CountSampTime=1.86011904761905e-08
      settings: SourceProductBaseCode=HD
  Multiply-Add : hdlsllib/HDL Operations/Multiply-Add  Function=c+(a.*b)  datatype=fixdt(1, 32, 16)  DoSatur=off  FMA=off
      settings: SourceProductName=HDL Coder  SourceProductBaseCode=HD
  Switch : Switch  Criteria=u2 ~= 0  Threshold=double(0)  OutDataTypeStr=fixdt(1, 32, 16)  SampleTime=1.86011904761905e-08
  Switch1 : Switch  Criteria=u2 ~= 0  Threshold=double(0)  OutDataTypeStr=fixdt(1, 16, 15)  SampleTime=1.86011904761905e-08
  Switch2 : Switch  Criteria=u2 ~= 0  Threshold=double(0)  OutDataTypeStr=fixdt(1, 16, 15)  SampleTime=1.86011904761905e-08
  dout : Outport
  vout : Outport  Port=2
  wires:
  Switch/1 -> Multiply-Add/3
  Delay1/1 -> Switch/3
  vin/1 -> HDL Counter/2, Switch2/2, Switch1/2
  start/1 -> Switch/2, HDL Counter/1
  gs/1 -> Switch2/1
  rx/1 -> Switch1/1
  Compare To Constant1/1 -> vout/1
  Constant/1 -> Switch/1
  Constant1/1 -> Switch2/3, Switch1/3
  HDL Counter/1 -> Compare To Constant1/1
  Multiply-Add/1 -> Delay1/1, dout/1
  Switch1/1 -> Multiply-Add/1
  Switch2/1 -> Multiply-Add/2

== system gm_ZynqBF_2tx_fpga/channel_estimator/peakdetect_ch1/correlator1/correlator_i_instance20 ==
  rx : Inport  OutDataTypeStr=fixdt(1, 16, 15)  PortDimensions=1  SampleTime=1.86011904761905e-08
  gs : Inport  Port=2  OutDataTypeStr=fixdt(1, 16, 15)  PortDimensions=1  SampleTime=1.86011904761905e-08
  start : Inport  Port=3  OutDataTypeStr=boolean  PortDimensions=1  SampleTime=1.86011904761905e-08
  vin : Inport  Port=4  OutDataTypeStr=boolean  PortDimensions=1  SampleTime=1.86011904761905e-08
  Compare To Constant1 : simulink/Logic and Bit Operations/Compare To Constant  relop===  const=fi(0,0,7,0,'hex','3f')  OutDataTypeStr=boolean
  Constant : Constant  Value=0  OutDataTypeStr=fixdt(1, 32, 16)  SampleTime=-1
  Constant1 : Constant  Value=0  OutDataTypeStr=fixdt(1, 16, 15)  SampleTime=-1
  Delay1 : Delay  DelayLength=double(1)  InitialCondition=0  InputProcessing=Inherited  SampleTime=1.86011904761905e-08
  HDL Counter : hdlsllib/Sources/HDL Counter  CountType=Free running  CountInit=double(0)  CountStep=double(1)  CountMax=25  CountFromType=Initial value  CountFrom=double(0)  CountResetPort=on  CountLoadPort=off  CountEnbPort=on  CountDirPort=off  CountDataType=Unsigned  CountWordLen=7  CountFracLen=0  CountSampTime=1.86011904761905e-08
      settings: SourceProductBaseCode=HD
  Multiply-Add : hdlsllib/HDL Operations/Multiply-Add  Function=c+(a.*b)  datatype=fixdt(1, 32, 16)  DoSatur=off  FMA=off
      settings: SourceProductName=HDL Coder  SourceProductBaseCode=HD
  Switch : Switch  Criteria=u2 ~= 0  Threshold=double(0)  OutDataTypeStr=fixdt(1, 32, 16)  SampleTime=1.86011904761905e-08
  Switch1 : Switch  Criteria=u2 ~= 0  Threshold=double(0)  OutDataTypeStr=fixdt(1, 16, 15)  SampleTime=1.86011904761905e-08
  Switch2 : Switch  Criteria=u2 ~= 0  Threshold=double(0)  OutDataTypeStr=fixdt(1, 16, 15)  SampleTime=1.86011904761905e-08
  dout : Outport
  vout : Outport  Port=2
  wires:
  Switch/1 -> Multiply-Add/3
  Delay1/1 -> Switch/3
  vin/1 -> HDL Counter/2, Switch2/2, Switch1/2
  start/1 -> Switch/2, HDL Counter/1
  gs/1 -> Switch2/1
  rx/1 -> Switch1/1
  Compare To Constant1/1 -> vout/1
  Constant/1 -> Switch/1
  Constant1/1 -> Switch2/3, Switch1/3
  HDL Counter/1 -> Compare To Constant1/1
  Multiply-Add/1 -> Delay1/1, dout/1
  Switch1/1 -> Multiply-Add/1
  Switch2/1 -> Multiply-Add/2

== system gm_ZynqBF_2tx_fpga/channel_estimator/peakdetect_ch1/correlator1/correlator_i_instance21 ==
  rx : Inport  OutDataTypeStr=fixdt(1, 16, 15)  PortDimensions=1  SampleTime=1.86011904761905e-08
  gs : Inport  Port=2  OutDataTypeStr=fixdt(1, 16, 15)  PortDimensions=1  SampleTime=1.86011904761905e-08
  start : Inport  Port=3  OutDataTypeStr=boolean  PortDimensions=1  SampleTime=1.86011904761905e-08
  vin : Inport  Port=4  OutDataTypeStr=boolean  PortDimensions=1  SampleTime=1.86011904761905e-08
  Compare To Constant1 : simulink/Logic and Bit Operations/Compare To Constant  relop===  const=fi(0,0,7,0,'hex','3f')  OutDataTypeStr=boolean
  Constant : Constant  Value=0  OutDataTypeStr=fixdt(1, 32, 16)  SampleTime=-1
  Constant1 : Constant  Value=0  OutDataTypeStr=fixdt(1, 16, 15)  SampleTime=-1
  Delay1 : Delay  DelayLength=double(1)  InitialCondition=0  InputProcessing=Inherited  SampleTime=1.86011904761905e-08
  HDL Counter : hdlsllib/Sources/HDL Counter  CountType=Free running  CountInit=double(0)  CountStep=double(1)  CountMax=25  CountFromType=Initial value  CountFrom=double(0)  CountResetPort=on  CountLoadPort=off  CountEnbPort=on  CountDirPort=off  CountDataType=Unsigned  CountWordLen=7  CountFracLen=0  CountSampTime=1.86011904761905e-08
      settings: SourceProductBaseCode=HD
  Multiply-Add : hdlsllib/HDL Operations/Multiply-Add  Function=c+(a.*b)  datatype=fixdt(1, 32, 16)  DoSatur=off  FMA=off
      settings: SourceProductName=HDL Coder  SourceProductBaseCode=HD
  Switch : Switch  Criteria=u2 ~= 0  Threshold=double(0)  OutDataTypeStr=fixdt(1, 32, 16)  SampleTime=1.86011904761905e-08
  Switch1 : Switch  Criteria=u2 ~= 0  Threshold=double(0)  OutDataTypeStr=fixdt(1, 16, 15)  SampleTime=1.86011904761905e-08
  Switch2 : Switch  Criteria=u2 ~= 0  Threshold=double(0)  OutDataTypeStr=fixdt(1, 16, 15)  SampleTime=1.86011904761905e-08
  dout : Outport
  vout : Outport  Port=2
  wires:
  Switch/1 -> Multiply-Add/3
  Delay1/1 -> Switch/3
  vin/1 -> HDL Counter/2, Switch2/2, Switch1/2
  start/1 -> Switch/2, HDL Counter/1
  gs/1 -> Switch2/1
  rx/1 -> Switch1/1
  Compare To Constant1/1 -> vout/1
  Constant/1 -> Switch/1
  Constant1/1 -> Switch2/3, Switch1/3
  HDL Counter/1 -> Compare To Constant1/1
  Multiply-Add/1 -> Delay1/1, dout/1
  Switch1/1 -> Multiply-Add/1
  Switch2/1 -> Multiply-Add/2

== system gm_ZynqBF_2tx_fpga/channel_estimator/peakdetect_ch1/correlator1/correlator_i_instance22 ==
  rx : Inport  OutDataTypeStr=fixdt(1, 16, 15)  PortDimensions=1  SampleTime=1.86011904761905e-08
  gs : Inport  Port=2  OutDataTypeStr=fixdt(1, 16, 15)  PortDimensions=1  SampleTime=1.86011904761905e-08
  start : Inport  Port=3  OutDataTypeStr=boolean  PortDimensions=1  SampleTime=1.86011904761905e-08
  vin : Inport  Port=4  OutDataTypeStr=boolean  PortDimensions=1  SampleTime=1.86011904761905e-08
  Compare To Constant1 : simulink/Logic and Bit Operations/Compare To Constant  relop===  const=fi(0,0,7,0,'hex','3f')  OutDataTypeStr=boolean
  Constant : Constant  Value=0  OutDataTypeStr=fixdt(1, 32, 16)  SampleTime=-1
  Constant1 : Constant  Value=0  OutDataTypeStr=fixdt(1, 16, 15)  SampleTime=-1
  Delay1 : Delay  DelayLength=double(1)  InitialCondition=0  InputProcessing=Inherited  SampleTime=1.86011904761905e-08
  HDL Counter : hdlsllib/Sources/HDL Counter  CountType=Free running  CountInit=double(0)  CountStep=double(1)  CountMax=25  CountFromType=Initial value  CountFrom=double(0)  CountResetPort=on  CountLoadPort=off  CountEnbPort=on  CountDirPort=off  CountDataType=Unsigned  CountWordLen=7  CountFracLen=0  CountSampTime=1.86011904761905e-08
      settings: SourceProductBaseCode=HD
  Multiply-Add : hdlsllib/HDL Operations/Multiply-Add  Function=c+(a.*b)  datatype=fixdt(1, 32, 16)  DoSatur=off  FMA=off
      settings: SourceProductName=HDL Coder  SourceProductBaseCode=HD
  Switch : Switch  Criteria=u2 ~= 0  Threshold=double(0)  OutDataTypeStr=fixdt(1, 32, 16)  SampleTime=1.86011904761905e-08
  Switch1 : Switch  Criteria=u2 ~= 0  Threshold=double(0)  OutDataTypeStr=fixdt(1, 16, 15)  SampleTime=1.86011904761905e-08
  Switch2 : Switch  Criteria=u2 ~= 0  Threshold=double(0)  OutDataTypeStr=fixdt(1, 16, 15)  SampleTime=1.86011904761905e-08
  dout : Outport
  vout : Outport  Port=2
  wires:
  Switch/1 -> Multiply-Add/3
  Delay1/1 -> Switch/3
  vin/1 -> HDL Counter/2, Switch2/2, Switch1/2
  start/1 -> Switch/2, HDL Counter/1
  gs/1 -> Switch2/1
  rx/1 -> Switch1/1
  Compare To Constant1/1 -> vout/1
  Constant/1 -> Switch/1
  Constant1/1 -> Switch2/3, Switch1/3
  HDL Counter/1 -> Compare To Constant1/1
  Multiply-Add/1 -> Delay1/1, dout/1
  Switch1/1 -> Multiply-Add/1
  Switch2/1 -> Multiply-Add/2

== system gm_ZynqBF_2tx_fpga/channel_estimator/peakdetect_ch1/correlator1/correlator_i_instance23 ==
  rx : Inport  OutDataTypeStr=fixdt(1, 16, 15)  PortDimensions=1  SampleTime=1.86011904761905e-08
  gs : Inport  Port=2  OutDataTypeStr=fixdt(1, 16, 15)  PortDimensions=1  SampleTime=1.86011904761905e-08
  start : Inport  Port=3  OutDataTypeStr=boolean  PortDimensions=1  SampleTime=1.86011904761905e-08
  vin : Inport  Port=4  OutDataTypeStr=boolean  PortDimensions=1  SampleTime=1.86011904761905e-08
  Compare To Constant1 : simulink/Logic and Bit Operations/Compare To Constant  relop===  const=fi(0,0,7,0,'hex','3f')  OutDataTypeStr=boolean
  Constant : Constant  Value=0  OutDataTypeStr=fixdt(1, 32, 16)  SampleTime=-1
  Constant1 : Constant  Value=0  OutDataTypeStr=fixdt(1, 16, 15)  SampleTime=-1
  Delay1 : Delay  DelayLength=double(1)  InitialCondition=0  InputProcessing=Inherited  SampleTime=1.86011904761905e-08
  HDL Counter : hdlsllib/Sources/HDL Counter  CountType=Free running  CountInit=double(0)  CountStep=double(1)  CountMax=25  CountFromType=Initial value  CountFrom=double(0)  CountResetPort=on  CountLoadPort=off  CountEnbPort=on  CountDirPort=off  CountDataType=Unsigned  CountWordLen=7  CountFracLen=0  CountSampTime=1.86011904761905e-08
      settings: SourceProductBaseCode=HD
  Multiply-Add : hdlsllib/HDL Operations/Multiply-Add  Function=c+(a.*b)  datatype=fixdt(1, 32, 16)  DoSatur=off  FMA=off
      settings: SourceProductName=HDL Coder  SourceProductBaseCode=HD
  Switch : Switch  Criteria=u2 ~= 0  Threshold=double(0)  OutDataTypeStr=fixdt(1, 32, 16)  SampleTime=1.86011904761905e-08
  Switch1 : Switch  Criteria=u2 ~= 0  Threshold=double(0)  OutDataTypeStr=fixdt(1, 16, 15)  SampleTime=1.86011904761905e-08
  Switch2 : Switch  Criteria=u2 ~= 0  Threshold=double(0)  OutDataTypeStr=fixdt(1, 16, 15)  SampleTime=1.86011904761905e-08
  dout : Outport
  vout : Outport  Port=2
  wires:
  Switch/1 -> Multiply-Add/3
  Delay1/1 -> Switch/3
  vin/1 -> HDL Counter/2, Switch2/2, Switch1/2
  start/1 -> Switch/2, HDL Counter/1
  gs/1 -> Switch2/1
  rx/1 -> Switch1/1
  Compare To Constant1/1 -> vout/1
  Constant/1 -> Switch/1
  Constant1/1 -> Switch2/3, Switch1/3
  HDL Counter/1 -> Compare To Constant1/1
  Multiply-Add/1 -> Delay1/1, dout/1
  Switch1/1 -> Multiply-Add/1
  Switch2/1 -> Multiply-Add/2

== system gm_ZynqBF_2tx_fpga/channel_estimator/peakdetect_ch1/correlator1/correlator_i_instance24 ==
  rx : Inport  OutDataTypeStr=fixdt(1, 16, 15)  PortDimensions=1  SampleTime=1.86011904761905e-08
  gs : Inport  Port=2  OutDataTypeStr=fixdt(1, 16, 15)  PortDimensions=1  SampleTime=1.86011904761905e-08
  start : Inport  Port=3  OutDataTypeStr=boolean  PortDimensions=1  SampleTime=1.86011904761905e-08
  vin : Inport  Port=4  OutDataTypeStr=boolean  PortDimensions=1  SampleTime=1.86011904761905e-08
  Compare To Constant1 : simulink/Logic and Bit Operations/Compare To Constant  relop===  const=fi(0,0,7,0,'hex','3f')  OutDataTypeStr=boolean
  Constant : Constant  Value=0  OutDataTypeStr=fixdt(1, 32, 16)  SampleTime=-1
  Constant1 : Constant  Value=0  OutDataTypeStr=fixdt(1, 16, 15)  SampleTime=-1
  Delay1 : Delay  DelayLength=double(1)  InitialCondition=0  InputProcessing=Inherited  SampleTime=1.86011904761905e-08
  HDL Counter : hdlsllib/Sources/HDL Counter  CountType=Free running  CountInit=double(0)  CountStep=double(1)  CountMax=25  CountFromType=Initial value  CountFrom=double(0)  CountResetPort=on  CountLoadPort=off  CountEnbPort=on  CountDirPort=off  CountDataType=Unsigned  CountWordLen=7  CountFracLen=0  CountSampTime=1.86011904761905e-08
      settings: SourceProductBaseCode=HD
  Multiply-Add : hdlsllib/HDL Operations/Multiply-Add  Function=c+(a.*b)  datatype=fixdt(1, 32, 16)  DoSatur=off  FMA=off
      settings: SourceProductName=HDL Coder  SourceProductBaseCode=HD
  Switch : Switch  Criteria=u2 ~= 0  Threshold=double(0)  OutDataTypeStr=fixdt(1, 32, 16)  SampleTime=1.86011904761905e-08
  Switch1 : Switch  Criteria=u2 ~= 0  Threshold=double(0)  OutDataTypeStr=fixdt(1, 16, 15)  SampleTime=1.86011904761905e-08
  Switch2 : Switch  Criteria=u2 ~= 0  Threshold=double(0)  OutDataTypeStr=fixdt(1, 16, 15)  SampleTime=1.86011904761905e-08
  dout : Outport
  vout : Outport  Port=2
  wires:
  Switch/1 -> Multiply-Add/3
  Delay1/1 -> Switch/3
  vin/1 -> HDL Counter/2, Switch2/2, Switch1/2
  start/1 -> Switch/2, HDL Counter/1
  gs/1 -> Switch2/1
  rx/1 -> Switch1/1
  Compare To Constant1/1 -> vout/1
  Constant/1 -> Switch/1
  Constant1/1 -> Switch2/3, Switch1/3
  HDL Counter/1 -> Compare To Constant1/1
  Multiply-Add/1 -> Delay1/1, dout/1
  Switch1/1 -> Multiply-Add/1
  Switch2/1 -> Multiply-Add/2
